simulink model "rtwdemo_codegenrpt"  (Simulink 7.6)
settings: Solver=FixedStepDiscrete  StartTime=0.0  StopTime=48  FixedStep=1  RelTol=1e-3  SampleTimeConstraint=STIndependent
PostLoadFcn:
  | INC=uint8(1);LIMIT=uint8(16);RESET=uint8(0);K=int32(2);
libraries: rtwdemowidgets x3
Description:
  | Documenting Generated Code
settings Model: Creator=The MathWorks Inc.  ParamWorkspaceSource=ReferencedWorkspace  CovMetricSettings=d  ExtModeTrigMode=oneshot  ExtModeArmWhenConnect=off  ExtModeAutoUpdateStatusClock=off
settings MATStruct: SampleTime=1  Offset=0  Priority=[41.0]
settings DataIOCC: LimitDataPoints=off  SaveFormat=StructureWithTime  SaveOutput=off  SaveTime=off  SignalLoggingName=sigsOut
settings OptimizationCC: InlineParams=on  InlineInvariantSignals=on  StateBitsets=on  DataBitsets=on  UseTempVars=on  EfficientFloat2IntCast=on  EfficientMapNaN2IntZero=off  BufferReusableBoundary=off
settings DebuggingCC: CheckExecutionContextPreStartOutputMsg=on  CheckExecutionContextRuntimeOutputMsg=on  SolverPrmCheckMsg=none  IntegerOverflowMsg=none  StrictBusMsg=ErrorOnBusTreatedAsVector
settings HardwareCC: ProdIntDivRoundTo=Zero  ProdEndianess=LittleEndian  ProdHWDeviceType=Generic->32-bit Embedded Processor  TargetHWDeviceType=Generic->32-bit Embedded Processor
settings ModelReferenceCC: UpdateModelReferenceTargets=IfOutOfDate
settings RTWCC: TLCOptions=-p0 -aWarnNonSaturatedBlocks=0  GenerateReport=on  RTWVerbose=off  ProcessScript=grt_make_rtw_hook  LaunchReport=on  IncludeERTFirstTime=on
settings CodeAppCC: ForceParamTrailComments=on
settings GRTTargetCC: TargetFcnLib=ansi_tfl_tmw.mat

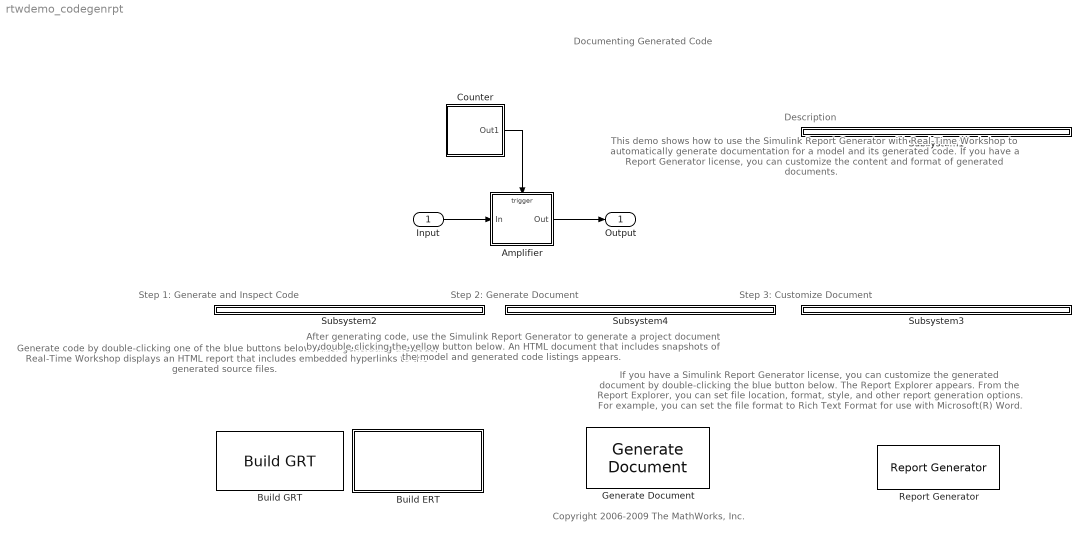
== system rtwdemo_codegenrpt ==
  note: Copyright 2006-2009 The MathWorks, Inc.
  note: Documenting Generated Code
  note: Generate code by double-clicking one of the
      | blue buttons below. After generating the code,
      | Real-Time Workshop displays an HTML report
      | that includes embedded hyperlinks to the
      | generated source files.
  note: Step 1: Generate and Inspect Code
  note: After generating code, use the Simulink Report
      | Generator to generate a project document by
      | double clicking the yellow button below. An
      | HTML document that includes snapshots of the
      | model and generated code listings appears.
  note: Step 2: Generate Document
  note: Description
  note: If you have a Simulink Report Generator license,
      | you can customize the generated document by
      | double-clicking the blue button below. The Report
      | Explorer appears. From the Report Explorer, you
      | can set file location, format, style, and other
      | report generation options. For example, you can
      | set the file format to Rich Text Format for use
      | with Microsoft(R) Word.
  note: Step 3: Customize Document
  note: This demo shows how to use the Simulink
      | Report Generator with Real-Time Workshop to
      | automatically generate documentation for a
      | model and its generated code. If you have a
      | Report Generator license, you can customize
      | the content and format of generated documents.
  Input : Inport  OutDataTypeStr=int32  PortDimensions=1
  Amplifier : Subsystem  TreatAsAtomicUnit=on
  Build ERT : Subsystem  mask{attrib_overrides={}}
      mask prompts: attrib_overrides "List of attributes to preserve (cell of strings):"
      mask help: Enter the attributes of the configuration set that you want preserved. Otherwise, the default configuration script will override your current settings.
      settings: OpenFcn=|
      | model=bdroot; overrides=get_param(gcb,'attrib_overrides');
      | try
      | 
      | rtwconfiguredemo(model,'noop',false,overrides);
      | 
      | set_param(model,'PurelyIntegerCode','on');
      | set_param(model,'SupportNonFinite','off');
      | set_param(model,'SupportComplex','off');
      | set_param(model,'SupportAbsoluteTime','off');
      | set_param(model,'SupportContinuousTime','off');
      | set_param(model,'SupportNonInlinedSFcns','off');
      | 
      | set_param(model','dirty','off');
      | 
      | rtwbuilddemomodel(model);
      | catch
      |   error(lasterr);
      | end
      |   clear model overrides;
      mask Display:
      | disp(['Generate Code Using\n',...
      | 	  'Real-Time Workshop\n',...
      | 	  'Embedded Coder\n'...
      | 	  '(double-click)'])
  Build GRT : rtwdemowidgets/Build GRT  SystemSampleTime=-1  attrib_overrides={}
  Counter : Subsystem
  Generate Document : rtwdemowidgets/Generate Document  SystemSampleTime=-1
  Report Generator : rtwdemowidgets/Report Generator  SystemSampleTime=-1
  Subsystem1 : Subsystem
      mask Description: Line
  Subsystem2 : Subsystem
      mask Description: Line
  Subsystem3 : Subsystem
      mask Description: Line
  Subsystem4 : Subsystem
      mask Description: Line
  Output : Outport
  wires:
  Input/1 -> Amplifier/1(In)
  Amplifier/1(Out) -> Output/1
  Counter/1(Out1) -> Amplifier/Trigger

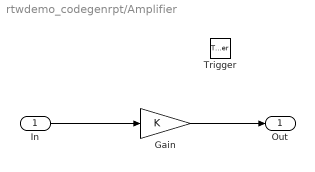
== system rtwdemo_codegenrpt/Amplifier ==
  In : Inport
  Trigger : TriggerPort
  Gain : Gain  Gain=K  OutDataTypeStr=Inherit: Same as input  ParamDataTypeStr=Inherit: Same as input
  Out : Outport  InitialOutput=0
  wires:
  In/1 -> Gain/1
  Gain/1 -> Out/1

== system rtwdemo_codegenrpt/Build ERT ==

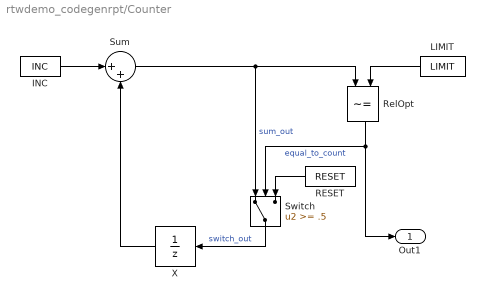
== system rtwdemo_codegenrpt/Counter ==
  INC : Constant  Value=INC
  LIMIT : Constant  Value=LIMIT
  RESET : Constant  Value=RESET
  RelOpt : RelationalOperator  Operator=~=  InputSameDT=on
  Sum : Sum  Inputs=|++  InputSameDT=on  OutDataTypeStr=Inherit: Same as first input
  Switch : Switch  Threshold=.5  InputSameDT=on
  X : UnitDelay  SampleTime=-1  StateIdentifier=X
  Out1 : Outport
  wires:
  INC/1 -> Sum/1
  X/1 -> Sum/2
  Switch/1 -> X/1  "switch_out"
  Sum/1 -> Switch/1, RelOpt/1  "sum_out"
  LIMIT/1 -> RelOpt/2
  RESET/1 -> Switch/3
  RelOpt/1 -> Switch/2, Out1/1  "equal_to_count"

== system rtwdemo_codegenrpt/Subsystem1 ==

== system rtwdemo_codegenrpt/Subsystem2 ==

== system rtwdemo_codegenrpt/Subsystem3 ==

== system rtwdemo_codegenrpt/Subsystem4 ==
